simulink model "SIP_Model"  (R2021a)
settings: Solver=ode1  StartTime=0.0  StopTime=60  FixedStep=0.002  RelTol=1e-3  EnableMultiTasking=on
undefined symbols (not defined in the file): g, HIL, J, K, K_AMP, l, mp, wcf, zetaf
libraries: quarc_library x7, simulink_extras x2, simulink x2
settings Model: ExtModeTrigDuration=50001  Creator=Mechatronics  LastModifiedBy=User
settings SolverCC: AlgebraicLoopSolver=TrustRegion  PositivePriorityOrder=on
settings DataIOCC: ReturnWorkspaceOutputs=off
settings DebuggingCC: SFMachineParentedDataDiag=warning  ArithmeticOperatorsInVariantConditions=warning
settings SFSimCC: SimUseLocalCustomCode=off  CustomCodeUndefinedFunction=UseInterfaceOnly
settings RTWCC: Description=QUARC Win64 Target Using Toolchain  SystemTargetFile=quarc_win64.tlc  TemplateMakefile=quarc_default_tmf  RTWUseLocalCustomCode=off  Toolchain=QUARC win64 | nmake (64-bit Windows)  BuildConfiguration=Faster Runs
settings CodeAppCC: StateflowObjectComments=on
settings STFCustomTargetCC: TargetLangStandard=C99 (ISO)  ConcurrentExecutionCompliant=on  SystemTargetFile=quarc_win64.tlc
settings GRTTargetCC: ParMdlRefBuildCompliant=off  CompOptLevelCompliant=off  CombineOutputUpdateFcns=off  MatFileLogging=off  CPPClassGenCompliant=off  GRTInterface=on  ExtMode=on  ExtModeMexFile=quarc_comm
settings ConfigComp: CovMetricSettings=dswe

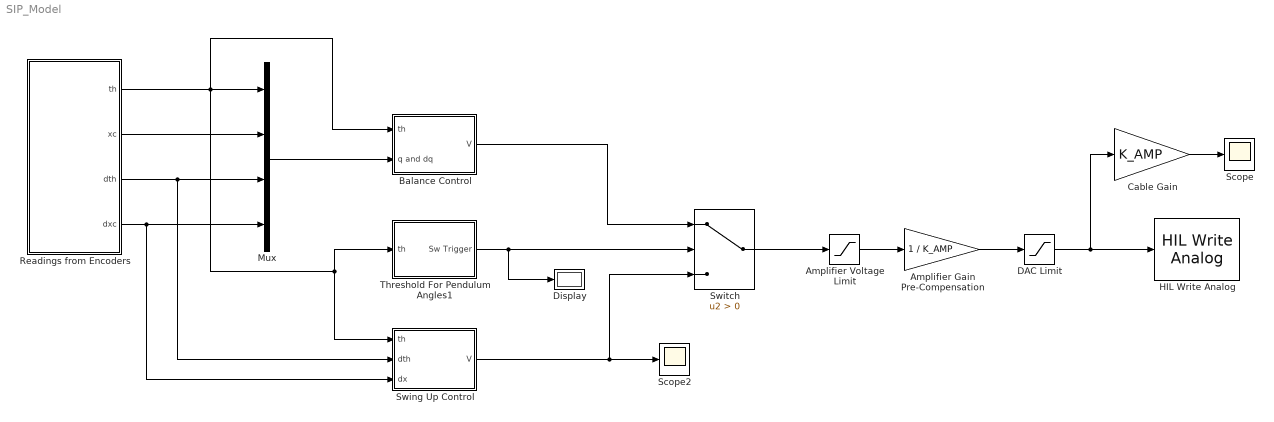
== system SIP_Model ==
  Amplifier Gain Pre-Compensation : Gain  Gain=1 / K_AMP  SaturateOnIntegerOverflow=on  OutDataTypeStr=Inherit: Same as input  ParamDataTypeStr=Inherit: Same as input
  Amplifier Voltage Limit : Saturate  UpperLimit=24  LowerLimit=-24
  Balance Control : Subsystem
  Cable Gain : Gain  Gain=K_AMP  SaturateOnIntegerOverflow=on  OutDataTypeStr=Inherit: Same as input  ParamDataTypeStr=Inherit: Same as input
  DAC Limit : Saturate  UpperLimit=10  LowerLimit=-10
  Display : Display
  HIL Write Analog : quarc_library/Data Acquisition/Generic/Immediate I//O/HIL Write Analog  object_name=HIL-1  channels=0  sample_time=-1  active=off  vector_input=off
  Mux : Mux
  Readings from Encoders : Subsystem
  Scope : Scope
  Scope2 : Scope
  Swing Up Control : Subsystem
  Switch : Switch  Criteria=u2 > Threshold
  Threshold For Pendulum Angles1 : Subsystem
  wires:
  Amplifier Voltage Limit/1 -> Amplifier Gain Pre-Compensation/1
  Threshold For Pendulum Angles1/1(Sw Trigger) -> Switch/2, Display/1
  Switch/1 -> Amplifier Voltage Limit/1
  DAC Limit/1 -> HIL Write Analog/1, Cable Gain/1
  Amplifier Gain Pre-Compensation/1 -> DAC Limit/1
  Cable Gain/1 -> Scope/1
  Readings from Encoders/1(th) -> Mux/1, Balance Control/1(th), Swing Up Control/1(th), Threshold For Pendulum Angles1/1(th)
  Readings from Encoders/2(xc) -> Mux/2
  Readings from Encoders/3(dth) -> Swing Up Control/2(dth), Mux/3
  Readings from Encoders/4(dxc) -> Swing Up Control/3(dx), Mux/4
  Balance Control/1(V) -> Switch/1
  Mux/1 -> Balance Control/2(q and dq)
  Swing Up Control/1(V) -> Scope2/1, Switch/3

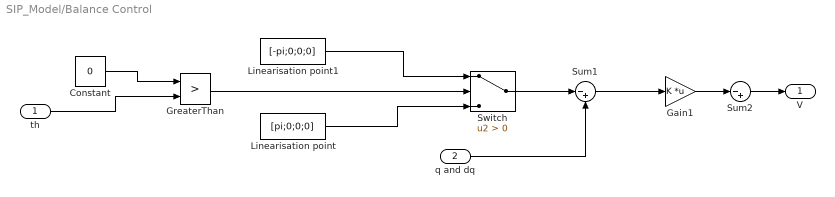
== system SIP_Model/Balance Control ==
  th : Inport
  q and dq : Inport  Port=2
  Constant : Constant  Value=0
  Gain1 : Gain  Gain=K  Multiplication=Matrix(K*u)
  GreaterThan : RelationalOperator  Operator=>  OutDataTypeStr=boolean  RndMeth=Simplest
  Linearisation point : Constant  Value=[pi;0;0;0]
  Linearisation point1 : Constant  Value=[-pi;0;0;0]
  Sum1 : Sum  Inputs=|-+
  Sum2 : Sum  Inputs=|-+
  Switch : Switch  Criteria=u2 > Threshold
  V : Outport
  wires:
  q and dq/1 -> Sum1/2
  Sum1/1 -> Gain1/1
  Gain1/1 -> Sum2/1
  Sum2/1 -> V/1
  Switch/1 -> Sum1/1
  Linearisation point/1 -> Switch/3
  GreaterThan/1 -> Switch/2
  Linearisation point1/1 -> Switch/1
  Constant/1 -> GreaterThan/1
  th/1 -> GreaterThan/2

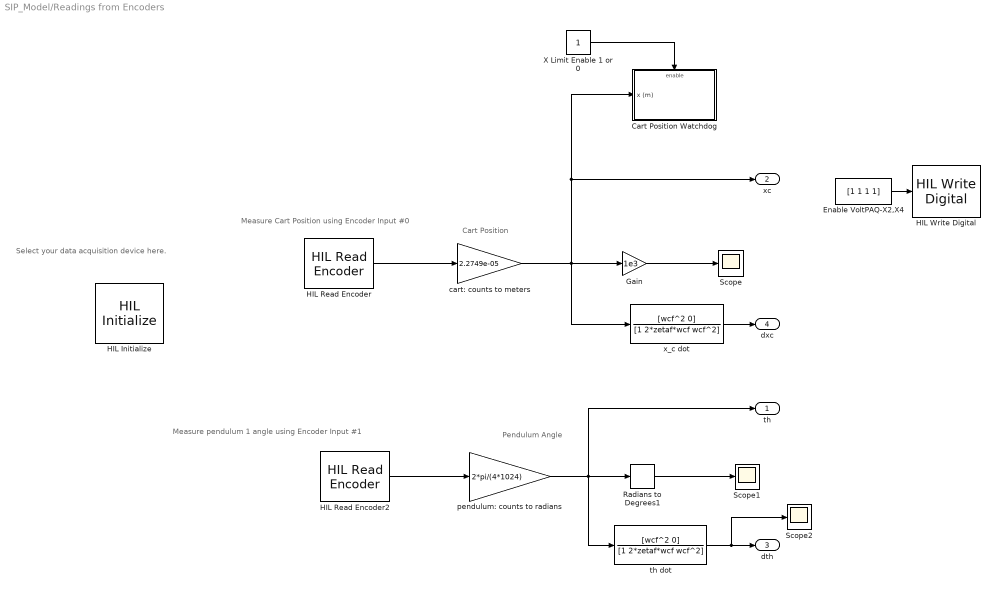
== system SIP_Model/Readings from Encoders ==
  note: Pendulum Angle
  note: Measure Cart Position using Encoder Input #0
  note: Cart Position
  note: Select your data acquisition device here.
  note: Measure pendulum 1 angle using Encoder Input #1
  Cart Position Watchdog : Subsystem  TreatAsAtomicUnit=on
  Enable VoltPAQ-X2,X4 : Constant  Value=[1 1 1 1]
  Gain : Gain  Gain=1e3
  HIL Initialize : quarc_library/Data Acquisition/Generic/Configuration/HIL Initialize  object_name=HIL-1  board_type=q8_usb  board_number=0  board_options=update_rate=normal  exclusive=off  active=off  hardware_clocks=[0:2]  clock_modes=[]  initial_clock_frequencies=[]  set_clock_params_at_start=off  set_clock_params_at_switch_in=off  set_clock_frequencies_at_start=off  set_clock_frequencies_at_switch_in=off  analog_input_channels=[0:7]  analog_input_configurations=[]  analog_input_maximums=10  analog_input_minimums=-10  set_analog_input_params_at_start=on  set_analog_input_params_at_switch_in=off  analog_output_channels=[0:7]  analog_output_maximums=10  analog_output_minimums=-10  initial_analog_outputs=[0]  final_analog_outputs=[0]  watchdog_analog_outputs=0  set_analog_output_params_at_start=on  set_analog_output_params_at_switch_in=off  set_analog_outputs_at_start=on  set_analog_outputs_at_switch_in=off  set_analog_outputs_at_terminate=on  set_analog_outputs_at_switch_out=off  set_analog_outputs_on_watchdog=off  digital_input_channels=[]  digital_output_channels=[0:7]  digital_output_configuration=[]  initial_digital_outputs=[0]  final_digital_outputs=[0]  watchdog_digital_outputs=[0]  set_digital_output_params_at_start=off  set_digital_output_params_at_switch_in=off  set_digital_outputs_at_start=on  set_digital_outputs_at_switch_in=off  set_digital_outputs_at_terminate=on  set_digital_outputs_at_switch_out=off  set_digital_outputs_on_watchdog=off  encoder_channels=[0:7]  quadrature=[4]  encoder_filter_frequency=[]  initial_encoder_counts=[0]  set_encoder_params_at_start=on  set_encoder_params_at_switch_in=off  set_encoder_counts_at_start=on  set_encoder_counts_at_switch_in=off  pwm_channels=[0:7]  pwm_modes=0  pwm_frequency=99.532799999999995e6/4095  pwm_configuration=[0]  pwm_alignment=[0]  pwm_polarity=[1]  pwm_leading_deadband=[0]  pwm_trailing_deadband=[0]  initial_pwm_outputs=[0]  final_pwm_outputs=[0]  watchdog_pwm_outputs=[0]  set_pwm_params_at_start=on  set_pwm_params_at_switch_in=off  set_pwm_outputs_at_start=on  set_pwm_outputs_at_switch_in=off  set_pwm_outputs_at_terminate=on  set_pwm_outputs_at_switch_out=off  set_pwm_outputs_on_watchdog=off  other_output_channels=[]  initial_other_outputs=[]  final_other_outputs=[]  watchdog_other_outputs=[]  set_other_outputs_at_start=off  set_other_outputs_at_switch_in=off  set_other_outputs_at_terminate=off  set_other_outputs_at_switch_out=off  set_other_outputs_on_watchdog=off
  HIL Read Encoder : quarc_library/Data Acquisition/Generic/Immediate I//O/HIL Read Encoder  object_name=HIL-1  channels=[0]  sample_time=qc_get_step_size  active=on  vector_output=off  data_type_mode=Inherit via back propagation  data_type=double
  HIL Read Encoder2 : quarc_library/Data Acquisition/Generic/Immediate I//O/HIL Read Encoder  object_name=HIL-1  channels=[1]  sample_time=qc_get_step_size  active=on  vector_output=off  data_type_mode=Inherit via back propagation  data_type=double
  HIL Write Digital : quarc_library/Data Acquisition/Generic/Immediate I//O/HIL Write Digital  object_name=HIL-1  channels=[0:3]  sample_time=-1  active=off  vector_input=on
      settings: SourceProductName=QUARC Targets
  Radians to Degrees1 : simulink_extras/Transformations/Radians to Degrees
  Scope : Scope
  Scope1 : Scope
  Scope2 : Scope
  X Limit Enable 1 or 0 : Constant
  cart: counts to meters : Gain  Gain=2.2749e-05  SaturateOnIntegerOverflow=on  OutDataTypeStr=Inherit: Same as input  ParamDataTypeStr=Inherit: Same as input
  pendulum: counts to radians : Gain  Gain=2*pi/(4*1024)  SaturateOnIntegerOverflow=on  OutDataTypeStr=Inherit: Same as input  ParamDataTypeStr=Inherit: Same as input
  th dot : TransferFcn  Numerator=[wcf^2 0]  Denominator=[1 2*zetaf*wcf wcf^2]
  x_c dot : TransferFcn  Numerator=[wcf^2 0]  Denominator=[1 2*zetaf*wcf wcf^2]
  th : Outport
  xc : Outport  Port=2
  dth : Outport  Port=3
  dxc : Outport  Port=4
  wires:
  HIL Read Encoder2/1 -> pendulum: counts to radians/1
  Enable VoltPAQ-X2,X4/1 -> HIL Write Digital/1
  pendulum: counts to radians/1 -> th/1, th dot/1, Radians to Degrees1/1
  Radians to Degrees1/1 -> Scope1/1
  HIL Read Encoder/1 -> cart: counts to meters/1
  Gain/1 -> Scope/1
  x_c dot/1 -> dxc/1
  th dot/1 -> Scope2/1, dth/1
  cart: counts to meters/1 -> Gain/1, Cart Position Watchdog/1(x (m)), xc/1, x_c dot/1
  X Limit Enable 1 or 0/1 -> Cart Position Watchdog/Enable

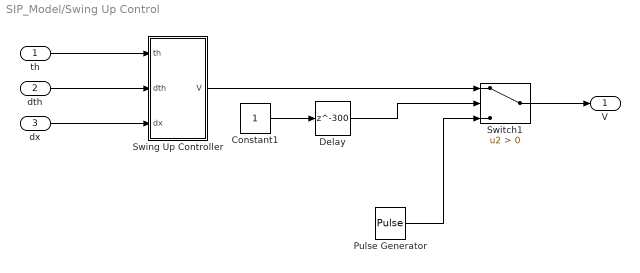
== system SIP_Model/Swing Up Control ==
  th : Inport
  dth : Inport  Port=2
  dx : Inport  Port=3
  Constant1 : Constant
  Delay : Delay  DelayLength=300  SampleTime=0.002
  Pulse Generator : DiscretePulseGenerator  PulseType=Time based  Amplitude=6  Period=100  PulseWidth=0.1
  Swing Up Controller : Subsystem
  Switch1 : Switch  Criteria=u2 > Threshold
  V : Outport
  wires:
  Delay/1 -> Switch1/2
  Pulse Generator/1 -> Switch1/3
  Constant1/1 -> Delay/1
  th/1 -> Swing Up Controller/1(th)
  Switch1/1 -> V/1
  Swing Up Controller/1(V) -> Switch1/1
  dth/1 -> Swing Up Controller/2(dth)
  dx/1 -> Swing Up Controller/3(dx)

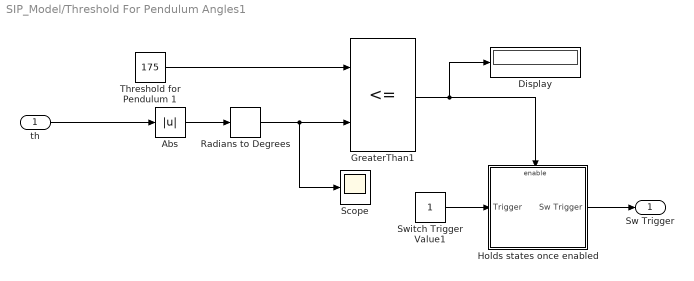
== system SIP_Model/Threshold For Pendulum Angles1 ==
  th : Inport
  Abs : Abs
  Display : Display
  GreaterThan1 : RelationalOperator  Operator=<=  OutDataTypeStr=boolean  RndMeth=Simplest
  Holds states once enabled : Subsystem  TreatAsAtomicUnit=on
  Radians to Degrees : simulink_extras/Transformations/Radians to Degrees
  Scope : Scope
  Switch Trigger Value1 : Constant
  Threshold for Pendulum 1 : Constant  Value=175
  Sw Trigger : Outport
  wires:
  GreaterThan1/1 -> Holds states once enabled/Enable, Display/1
  Holds states once enabled/1(Sw Trigger) -> Sw Trigger/1
  Switch Trigger Value1/1 -> Holds states once enabled/1(Trigger)
  Threshold for Pendulum 1/1 -> GreaterThan1/1
  Abs/1 -> Radians to Degrees/1
  Radians to Degrees/1 -> Scope/1, GreaterThan1/2
  th/1 -> Abs/1

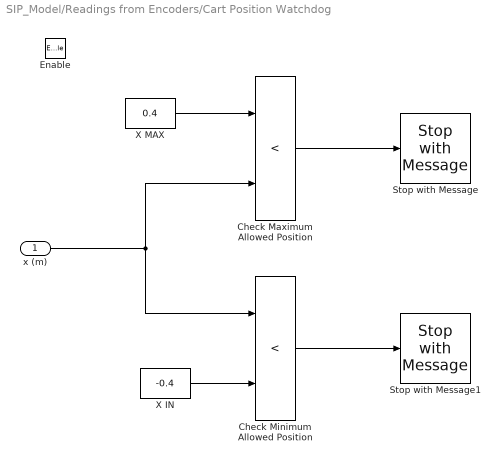
== system SIP_Model/Readings from Encoders/Cart Position Watchdog ==
  x (m) : Inport
  Enable : EnablePort
  Check Maximum Allowed Position : RelationalOperator  Operator=<  RndMeth=Nearest  InputSameDT=on
  Check Minimum Allowed Position : RelationalOperator  Operator=<  RndMeth=Nearest  InputSameDT=on
  Stop with Message : quarc_library/Sinks/Error Handling/Stop with Message  message_type=Fixed error message  message_icon=Warning  message=Maximum Cart Limit Reached.
  Stop with Message1 : quarc_library/Sinks/Error Handling/Stop with Message  message_type=Fixed error message  message_icon=Warning  message=Minimum Cart Limit Reached.
  X IN : Constant  Value=-0.4
  X MAX : Constant  Value=0.4
  wires:
  X MAX/1 -> Check Maximum Allowed Position/1
  Check Minimum Allowed Position/1 -> Stop with Message1/1
  X IN/1 -> Check Minimum Allowed Position/2
  x (m)/1 -> Check Maximum Allowed Position/2, Check Minimum Allowed Position/1
  Check Maximum Allowed Position/1 -> Stop with Message/1

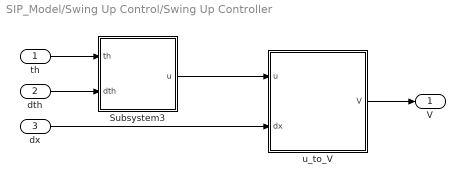
== system SIP_Model/Swing Up Control/Swing Up Controller ==
  th : Inport
  dth : Inport  Port=2
  dx : Inport  Port=3
  Subsystem3 : Subsystem
  u_to_V : MATLAB Function  TreatAsAtomicUnit=on
  V : Outport
  wires:
  th/1 -> Subsystem3/1(th)
  Subsystem3/1(u) -> u_to_V/1(u)
  dth/1 -> Subsystem3/2(dth)
  u_to_V/1(V) -> V/1
  dx/1 -> u_to_V/2(dx)

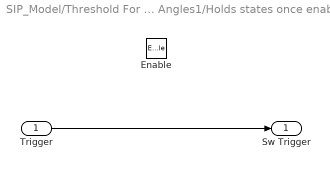
== system SIP_Model/Threshold For Pendulum Angles1/Holds states once enabled ==
  Trigger : Inport  OutDataTypeStr=double
  Enable : EnablePort
  Sw Trigger : Outport  OutDataTypeStr=double  InitialOutput=[0]
  wires:
  Trigger/1 -> Sw Trigger/1

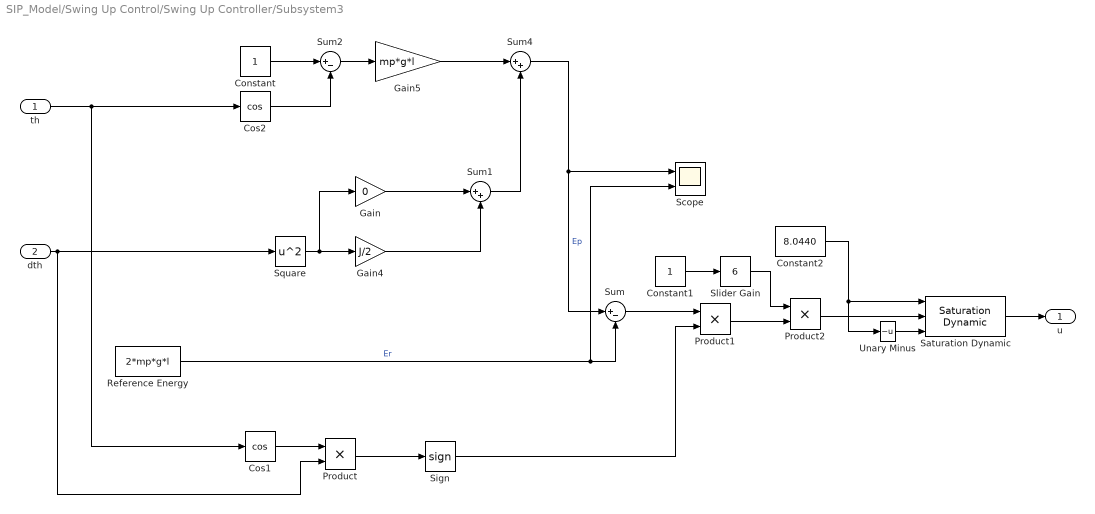
== system SIP_Model/Swing Up Control/Swing Up Controller/Subsystem3 ==
  th : Inport
  dth : Inport  Port=2
  Constant : Constant
  Constant1 : Constant
  Constant2 : Constant  Value=8.0440
  Cos1 : Trigonometry  Operator=cos
  Cos2 : Trigonometry  Operator=cos
  Gain : Gain  Gain=0
  Gain4 : Gain  Gain=J/2
  Gain5 : Gain  Gain=mp*g*l
  Product : Product
  Product1 : Product
  Product2 : Product
  Reference Energy : Constant  Value=2*mp*g*l
  Saturation Dynamic : simulink/Discontinuities/Saturation Dynamic  OutMin=[]  OutMax=[]  OutDataTypeStr=Inherit: Same as second input  OutDataType=fixdt(1, 16)  OutScaling=2^-10  DoSatur=off
  Scope : Scope  NumInputPorts=2
  Sign : Signum
  Slider Gain : simulink/Math Operations/Slider Gain  gain=6  low=0  high=10
  Square : Math  Operator=square  SaturateOnIntegerOverflow=on
  Sum : Sum  Inputs=|+-
  Sum1 : Sum  Inputs=|++
  Sum2 : Sum  Inputs=|+-
  Sum4 : Sum  Inputs=|++
  Unary Minus : UnaryMinus
  u : Outport
  wires:
  Gain5/1 -> Sum4/1
  Product1/1 -> Product2/2
  Sum1/1 -> Sum4/2
  Square/1 -> Gain/1, Gain4/1
  Gain4/1 -> Sum1/2
  dth/1 -> Square/1, Product/2
  Sum2/1 -> Gain5/1
  Cos1/1 -> Product/1
  Slider Gain/1 -> Product2/1
  Constant/1 -> Sum2/1
  Cos2/1 -> Sum2/2
  Constant1/1 -> Slider Gain/1
  th/1 -> Cos1/1, Cos2/1
  Reference Energy/1 -> Scope/2, Sum/2  "Er"
  Sum4/1 -> Sum/1, Scope/1  "Ep"
  Sum/1 -> Product1/1
  Gain/1 -> Sum1/1
  Product/1 -> Sign/1
  Product2/1 -> Saturation Dynamic/2
  Saturation Dynamic/1 -> u/1
  Constant2/1 -> Saturation Dynamic/1, Unary Minus/1
  Unary Minus/1 -> Saturation Dynamic/3
  Sign/1 -> Product1/2

== matlab function SIP_Model/Swing Up Control/Swing Up Controller/u_to_V ==
  data: u input; dx input; V output
function V = u_to_V(u,dx)
%#codegen

%    This function was generated by the Symbolic Math Toolbox version 8.7.
%    26-Oct-2022 11:43:40

mc = 0.57;

R_m = 2.6; 
k_t = 0.00767;
n_m = 1;
k_m = 0.00767;
K_g = 3.71;
n_g = 1;
r_mp = 6.35*10^(-3);

V = (K_g.*dx.*k_m)./r_mp+(R_m.*mc.*r_mp.*u)./(K_g.*k_t.*n_g.*n_m);
